simulink model "AUV_PID_Model_Stable"  (R2021a)
settings: Solver=ode45  StartTime=0.0  StopTime=30  MaxStep=0.01  RelTol=1e-4  AbsTol=1e-6
libraries: pid_lib x1
settings Model: Creator=opsip  LastModifiedBy=opsip

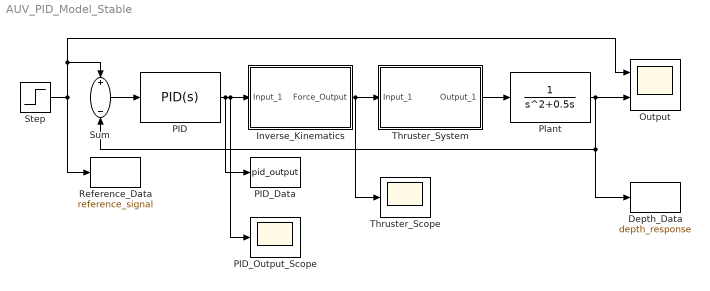
== system AUV_PID_Model_Stable ==
  Depth_Data : ToWorkspace  VariableName=depth_response  SampleTime=-1
  Inverse_Kinematics : Subsystem
  Output : Scope  NumInputPorts=2
  PID : pid_lib/PID Controller  Controller=PID  Form=Parallel  TimeDomain=Continuous-time  UseExternalTs=off  SampleTime=-1  IntegratorMethod=Forward Euler  FilterMethod=Forward Euler  ControllerParametersSource=internal  P=0.62  I=0.003  D=1.34  UseFilter=on  N=100  TunerSelectOption=Transfer Function Based (PID Tuner App)  InitialConditionSource=internal  InitialConditionForIntegrator=0  InitialConditionForFilter=0  DifferentiatorICPrevScaledInput=0  ExternalReset=none  TrackingMode=off  Kt=1  LimitOutput=off  SatLimitsSource=internal  UpperSaturationLimit=inf  LowerSaturationLimit=-inf  LinearizeAsGain=on  AntiWindupMode=none  Kb=1  POutMin=[]  POutMax=[]  IOutMin=[]  IOutMax=[]  DOutMin=[]  DOutMax=[]  NOutMin=[]  NOutMax=[]  SumOutMin=[]  SumOutMax=[]  SaturationOutMin=[]  SaturationOutMax=[]  PParamMin=[]  PParamMax=[]  IParamMin=[]  IParamMax=[]  DParamMin=[]  DParamMax=[]  NParamMin=[]  NParamMax=[]  KbParamMin=[]  KbParamMax=[]  KtParamMin=[]  KtParamMax=[]  KbOutMin=[]  KbOutMax=[]  KtOutMin=[]  KtOutMax=[]  IntegratorOutMin=[]  IntegratorOutMax=[]  FilterOutMin=[]  FilterOutMax=[]  SumI1OutMin=[]  SumI1OutMax=[]  SumI2OutMin=[]  SumI2OutMax=[]  SumI3OutMin=[]  SumI3OutMax=[]  SumI4OutMin=[]  SumI4OutMax=[]  SumDOutMin=[]  SumDOutMax=[]  DifferentiatorOutMin=[]  DifferentiatorOutMax=[]  FilterDiffOutCoefMin=[]  FilterDiffOutCoefMax=[]  ReciprocalOutMin=[]  ReciprocalOutMax=[]  SumDenOutMin=[]  SumDenOutMax=[]  SumNumOutMin=[]  SumNumOutMax=[]  DivideOutMin=[]  DivideOutMax=[]  UdiffTsProdOutMin=[]  UdiffTsProdOutMax=[]  NTsProdOutMin=[]  NTsProdOutMax=[]  UintegralTsProdOutMin=[]  UintegralTsProdOutMax=[]  UngainTsProdOutMin=[]  UngainTsProdOutMax=[]  IntegratorContinuousStateAttributes=''  IntegratorStateMustResolveToSignalObject=off  IntegratorRTWStateStorageClass=Auto  FilterContinuousStateAttributes=''  FilterStateMustResolveToSignalObject=off  FilterRTWStateStorageClass=Auto  ParallelPVariant=InternalParameters  IdealPVariant=Disabled  IVariant=InternalParameters  DVariant=InternalParameters  IntegratorVariant=Continuous  SatVariant=Disabled  AWVariant=Passthrough  PCopyVariant=Disabled  TRVariant=Disabled  FdbkBlocksVariant=Forward  IdealPFdbkVariant=Disabled  SatFdbkVariant=Disabled  DerivativeFilterVariant=ContFilter  NVariant=InternalParameters  NCopyVariant=Disabled  FilterICVariant=InternalICsFilter  IntegratorICVariant=InternalICs  ExternalResetVariant=Disabled  TRSumVariant=Passthrough  SumFdbkVariant=Disabled  SumVariant=Sum_PID  TsampFilterVariant=InternalTs  TsampNgainVariant=Passthrough  TsampIntegralVariant=Passthrough  ExternalSaturationOutDataTypeStr=Inherit: Same as second input
  PID_Data : ToWorkspace  VariableName=pid_output  SampleTime=-1
  PID_Output_Scope : Scope
  Plant : TransferFcn  Numerator=1  Denominator=[1 0.5 0]
  Reference_Data : ToWorkspace  VariableName=reference_signal  SampleTime=-1
  Step : Step  Time=2  After=10  SampleTime=0
  Sum : Sum  Inputs=+-
  Thruster_Scope : Scope
  Thruster_System : Subsystem
  wires:
  Step/1 -> Reference_Data/1, Sum/1, Output/1
  Sum/1 -> PID/1
  PID/1 -> Inverse_Kinematics/1(Input_1), PID_Output_Scope/1, PID_Data/1
  Inverse_Kinematics/1(Force_Output) -> Thruster_System/1(Input_1), Thruster_Scope/1
  Thruster_System/1(Output_1) -> Plant/1
  Plant/1 -> Sum/2, Depth_Data/1, Output/2

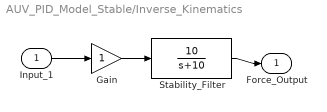
== system AUV_PID_Model_Stable/Inverse_Kinematics ==
  Input_1 : Inport
  Gain : Gain
  Stability_Filter : TransferFcn  Numerator=10  Denominator=[1 10]
  Force_Output : Outport
  wires:
  Input_1/1 -> Gain/1
  Gain/1 -> Stability_Filter/1
  Stability_Filter/1 -> Force_Output/1

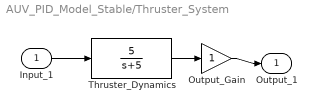
== system AUV_PID_Model_Stable/Thruster_System ==
  Input_1 : Inport
  Output_Gain : Gain
  Thruster_Dynamics : TransferFcn  Numerator=5  Denominator=[1 5]
  Output_1 : Outport
  wires:
  Input_1/1 -> Thruster_Dynamics/1
  Thruster_Dynamics/1 -> Output_Gain/1
  Output_Gain/1 -> Output_1/1
